simulink model "sf_msg_traffic_light"  (R2017b)
settings: Solver=FixedStepDiscrete  StartTime=0.0  StopTime=inf  FixedStep=.2  RelTol=1e-3  EnableMultiTasking=on
PostLoadFcn:
  | tl_gui('init', bdroot);
InitFcn:
  | tl_gui('reset', bdroot);
libraries: sf_msg_traffic_light_lib x6
CloseFcn:
  | tl_gui('close');
settings Model: Creator=The MathWorks, Inc.  LastModifiedBy=bea
settings DataIOCC: LimitDataPoints=on  SaveOutput=off  SignalLogging=off  DSMLogging=off  SaveTime=off
settings OptimizationCC: LifeSpan=inf
settings DebuggingCC: AllowSymbolicDim=off  SFUnexpectedBacktrackingDiag=warning  SFNoUnconditionalDefaultTransitionDiag=warning  SFExecutionAtInitializationDiag=none
settings HardwareCC: ProdBitPerPointer=32  ProdBitPerSizeT=32  ProdBitPerPtrDiffT=32  ProdLargestAtomicFloat=None  ProdIntDivRoundTo=Undefined  ProdEndianess=Unspecified  ProdWordSize=32  ProdHWDeviceType=32-bit Generic
settings ModelReferenceCC: PropagateSignalLabelsOutOfModel=off
settings RTWCC: GenCodeOnly=on  Description=Generic Real-Time Target  GenerateReport=on  LaunchReport=on
settings CodeAppCC: StateflowObjectComments=on
settings GRTTargetCC: TargetLangStandard=C89/C90 (ANSI)  UtilityFuncGeneration=Shared location  GeneratePreprocessorConditionals=Disable all
settings ConfigComp: CovMetricSettings=dw  CovHtmlReporting=on  CovSaveCumulativeToWorkspaceVar=on  CovSaveSingleToWorkspaceVar=on  CovExternalEMLEnable=off

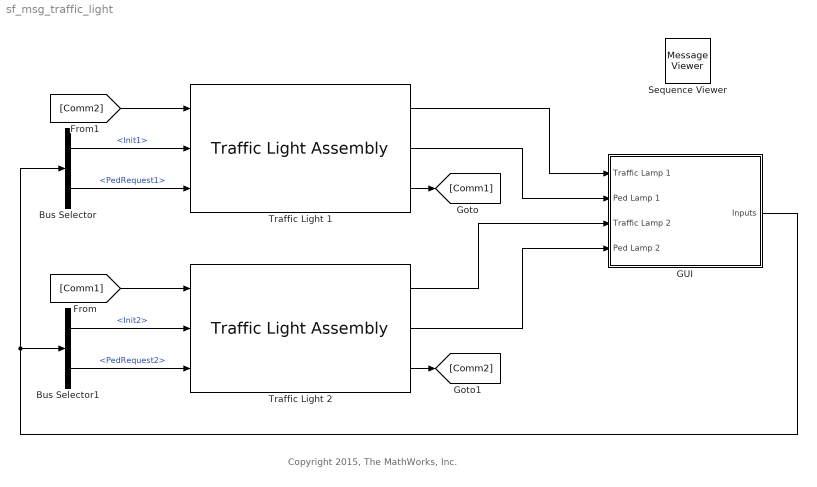
== system sf_msg_traffic_light ==
  note: Copyright 2015, The MathWorks, Inc.
  Bus Selector : BusSelector  OutputSignals=Init1,PedRequest1
  Bus Selector1 : BusSelector  OutputSignals=Init2,PedRequest2
  GUI : Subsystem
  Sequence Viewer : MessageViewer
  Traffic Light 1 : sf_msg_traffic_light_lib/Traffic Light Assembly
      settings: SourceProductName=Stateflow  SourceProductBaseCode=SF
  Traffic Light 2 : sf_msg_traffic_light_lib/Traffic Light Assembly
      settings: SourceProductName=Stateflow  SourceProductBaseCode=SF
  wires:
  Traffic Light 2/2 -> GUI/4(Ped Lamp 2)
  Traffic Light 2/1 -> GUI/3(Traffic Lamp 2)
  Traffic Light 1/2 -> GUI/2(Ped Lamp 1)
  Traffic Light 1/1 -> GUI/1(Traffic Lamp 1)
  Bus Selector/1 -> Traffic Light 1/2  "<Init1>"
  Bus Selector/2 -> Traffic Light 1/3  "<PedRequest1>"
  Bus Selector1/1 -> Traffic Light 2/2  "<Init2>"
  Bus Selector1/2 -> Traffic Light 2/3  "<PedRequest2>"
  GUI/1(Inputs) -> Bus Selector1/1, Bus Selector/1
  Traffic Light 1/3 -> [Comm1]
  Traffic Light 2/3 -> [Comm2]
  [Comm2] -> Traffic Light 1/1
  [Comm1] -> Traffic Light 2/1

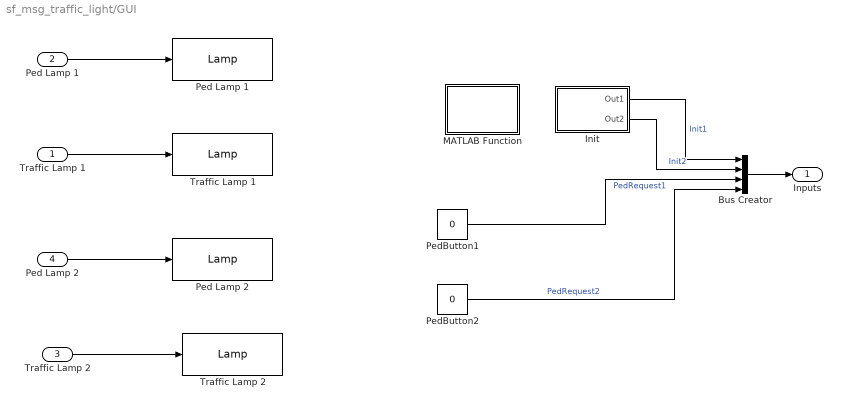
== system sf_msg_traffic_light/GUI ==
  Traffic Lamp 1 : Inport
  Ped Lamp 1 : Inport  Port=2
  Traffic Lamp 2 : Inport  Port=3
  Ped Lamp 2 : Inport  Port=4
  " Ped Lamp 1" : sf_msg_traffic_light_lib/ Lamp  LampSelect=Ped Lamp 1
      settings: SourceProductName=Stateflow  SourceProductBaseCode=SF
  " Ped Lamp 2" : sf_msg_traffic_light_lib/ Lamp  LampSelect=Ped Lamp 2
      settings: SourceProductName=Stateflow  SourceProductBaseCode=SF
  " Traffic Lamp 1" : sf_msg_traffic_light_lib/ Lamp  LampSelect=Traffic Lamp 1
      settings: SourceProductName=Stateflow  SourceProductBaseCode=SF
  " Traffic Lamp 2" : sf_msg_traffic_light_lib/ Lamp  LampSelect=Traffic Lamp 2
      settings: SourceProductName=Stateflow  SourceProductBaseCode=SF
  Bus Creator : BusCreator  Inputs=4
  Init : Subsystem
  MATLAB Function : MATLAB Function  TreatAsAtomicUnit=on
  PedButton1 : Constant  Value=0
  PedButton2 : Constant  Value=0
  Inputs : Outport
  wires:
  Init/1(Out1) -> Bus Creator/1  "Init1"
  Init/2(Out2) -> Bus Creator/2  "Init2"
  Bus Creator/1 -> Inputs/1
  Traffic Lamp 2/1 -> " Traffic Lamp 2"/1
  Ped Lamp 2/1 -> " Ped Lamp 2"/1
  Traffic Lamp 1/1 -> " Traffic Lamp 1"/1
  Ped Lamp 1/1 -> " Ped Lamp 1"/1
  PedButton1/1 -> Bus Creator/3  "PedRequest1"
  PedButton2/1 -> Bus Creator/4  "PedRequest2"

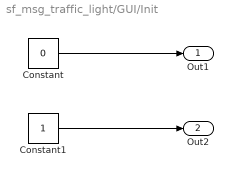
== system sf_msg_traffic_light/GUI/Init ==
  Constant : Constant  Value=0
  Constant1 : Constant
  Out1 : Outport
  Out2 : Outport  Port=2
  wires:
  Constant/1 -> Out1/1
  Constant1/1 -> Out2/1

== matlab function sf_msg_traffic_light/GUI/MATLAB Function ==
function pace()
pause(0.2);
